simulink model "BIM_3phaseModel_MidInject_DPNV"  (R2022b)
settings: Solver=VariableStepAuto  StartTime=0.0  StopTime=3  RelTol=1e-3
values from neighbouring files (symbols this model uses):
  Ad_s1_s = 0.730402691048646    (= 0.730402691049)    [BIM_init.m]
  Ad_t_s = 0.881911378298176    (= 0.881911378298)    [BIM_init.m]
  Ap_s1_s = 0.975904794542392    (= 0.975904794542)    [BIM_init.m]
  Ap_t_s = 0.995669127615556    (= 0.995669127616)    [BIM_init.m]
  Bd_s1_s = 0.269597308951354    (= 0.269597308951)    [BIM_init.m]
  Bd_t_s = 0.118088621701824    (= 0.118088621702)    [BIM_init.m]
  Bp_s1_s = 0.269597308951354    (= 0.269597308951)    [BIM_init.m]
  Bp_t_s = 0.118088621701824    (= 0.118088621702)    [BIM_init.m]
  Ctr_v_Ki = Ctr_v_Kp*0.1    (= 0.1)    [BIM_init.m]
  Ctr_v_Kp = 1    [BIM_init.m]
  L_m = 5.02e-3    (= 0.00502)    [BIM_init.m]
  L_r = L_m + L_sigma_r    (= 0.00576)    [BIM_init.m]
  m_rotor = 1.5    [BIM_init.m]
  PolePair = 1    [BIM_init.m]
  r_s1_s = 2*R_s    (= 1)    [BIM_init.m]
  r_t_s = R_s/2    (= 0.25)    [BIM_init.m]
  T = 1/fsw    (= 0.0001)    [BIM_init.m]
  tau_r = 0.012255319148936    (= 0.0122553191489)    [BIM_init.m]
  Ts = 1/fsw    (= 0.0001)    [BIM_init.m]
undefined symbols (not defined in the file or in its folder): plecs, sigbuilder_block
libraries: spsabctodq0Lib x8, spsdq0toabcLib x4
(part 2 of 2)

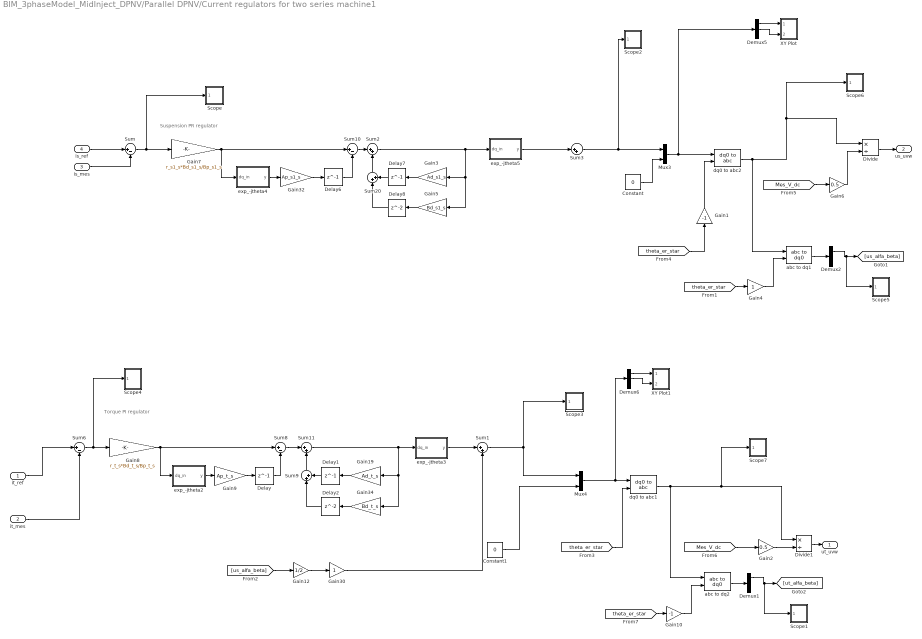
== system BIM_3phaseModel_MidInject_DPNV/Parallel DPNV/Current regulators for two series machine1 ==
  note: Suspension PR regulator
  note: Torque PI regulator
  it_ref : Inport  PortDimensions=2
  it_mes : Inport  Port=2  PortDimensions=2
  is_mes : Inport  Port=3  PortDimensions=2
  is_ref : Inport  Port=4  PortDimensions=2
  Constant : Constant  Value=0
  Constant1 : Constant  Value=0
  Delay{,1,6..7} (4 alike) : Delay  DelayLength=1  SampleTime=Ts
  Delay2 : Delay  SampleTime=Ts
  Delay8 : Delay  SampleTime=Ts
  Demux1 : Demux  Outputs=[2 1]
  Demux2 : Demux  Outputs=[2 1]
  Demux5 : Demux  Outputs=3
  Demux6 : Demux  Outputs=3
  Divide : Product  Inputs=*/
  Divide1 : Product  Inputs=*/
  Gain1 : Gain  Gain=-1
  Gain10 : Gain  Gain=-1
  Gain12 : Gain  Gain=1/2
  Gain19 : Gain  Gain=Ad_t_s
  Gain2 : Gain  Gain=0.5
  Gain3 : Gain  Gain=Ad_s1_s
  Gain30 : Gain
  Gain32 : Gain  Gain=Ap_s1_s
  Gain34 : Gain  Gain=Bd_t_s
  Gain4 : Gain
  Gain5 : Gain  Gain=Bd_s1_s
  Gain6 : Gain  Gain=0.5
  Gain7 : Gain  Gain=r_s1_s*Bd_s1_s/Bp_s1_s
  Gain8 : Gain  Gain=r_t_s*Bd_t_s/Bp_t_s
  Gain9 : Gain  Gain=Ap_t_s
  Mux3 : Mux  Inputs=[2 1]
  Mux4 : Mux  Inputs=[2 1]
  Scope : Subsystem  LoadFcn=plecs('sl', 300);  InitFcn=plecs('sl', 314);  StartFcn=plecs('sl', 308);  StopFcn=plecs('sl', 309);  mask{Settings=<binary blob, 232 chars, not shown>}
      mask init:
      | plecs('sl', 315);
      settings: CopyFcn=plecs('sl', 303);  DeleteFcn=plecs('sl', 305);  UndoDeleteFcn=plecs('sl', 306);  PreSaveFcn=plecs('sl', 311);  NameChangeFcn=plecs('sl', 310);  DestroyFcn=plecs('sl', 307);  OpenFcn=plecs('sl', 302);  ErrorFcn=plerrorfcn
      mask Display: plot([0.1 0.9 0.9 0.1 0.1], [0.9 0.9 0.5 0.5 0.9])
  Scope1 : Subsystem  LoadFcn=plecs('sl', 300);  InitFcn=plecs('sl', 314);  StartFcn=plecs('sl', 308);  StopFcn=plecs('sl', 309);  mask{Settings=<binary blob, 232 chars, not shown>}
      mask init:
      | plecs('sl', 315);
      settings: CopyFcn=plecs('sl', 303);  DeleteFcn=plecs('sl', 305);  UndoDeleteFcn=plecs('sl', 306);  PreSaveFcn=plecs('sl', 311);  NameChangeFcn=plecs('sl', 310);  DestroyFcn=plecs('sl', 307);  OpenFcn=plecs('sl', 302);  ErrorFcn=plerrorfcn
      mask Display: plot([0.1 0.9 0.9 0.1 0.1], [0.9 0.9 0.5 0.5 0.9])
  Scope2 : Subsystem  LoadFcn=plecs('sl', 300);  InitFcn=plecs('sl', 314);  StartFcn=plecs('sl', 308);  StopFcn=plecs('sl', 309);  mask{Settings=<binary blob, 232 chars, not shown>}
      mask init:
      | plecs('sl', 315);
      settings: CopyFcn=plecs('sl', 303);  DeleteFcn=plecs('sl', 305);  UndoDeleteFcn=plecs('sl', 306);  PreSaveFcn=plecs('sl', 311);  NameChangeFcn=plecs('sl', 310);  DestroyFcn=plecs('sl', 307);  OpenFcn=plecs('sl', 302);  ErrorFcn=plerrorfcn
      mask Display: plot([0.1 0.9 0.9 0.1 0.1], [0.9 0.9 0.5 0.5 0.9])
  Scope3 : Subsystem  LoadFcn=plecs('sl', 300);  InitFcn=plecs('sl', 314);  StartFcn=plecs('sl', 308);  StopFcn=plecs('sl', 309);  mask{Settings=<binary blob, 232 chars, not shown>}
      mask init:
      | plecs('sl', 315);
      settings: CopyFcn=plecs('sl', 303);  DeleteFcn=plecs('sl', 305);  UndoDeleteFcn=plecs('sl', 306);  PreSaveFcn=plecs('sl', 311);  NameChangeFcn=plecs('sl', 310);  DestroyFcn=plecs('sl', 307);  OpenFcn=plecs('sl', 302);  ErrorFcn=plerrorfcn
      mask Display: plot([0.1 0.9 0.9 0.1 0.1], [0.9 0.9 0.5 0.5 0.9])
  Scope4 : Subsystem  LoadFcn=plecs('sl', 300);  InitFcn=plecs('sl', 314);  StartFcn=plecs('sl', 308);  StopFcn=plecs('sl', 309);  mask{Settings=<binary blob, 232 chars, not shown>}
      mask init:
      | plecs('sl', 315);
      settings: CopyFcn=plecs('sl', 303);  DeleteFcn=plecs('sl', 305);  UndoDeleteFcn=plecs('sl', 306);  PreSaveFcn=plecs('sl', 311);  NameChangeFcn=plecs('sl', 310);  DestroyFcn=plecs('sl', 307);  OpenFcn=plecs('sl', 302);  ErrorFcn=plerrorfcn
      mask Display: plot([0.1 0.9 0.9 0.1 0.1], [0.9 0.9 0.5 0.5 0.9])
  Scope5 : Subsystem  LoadFcn=plecs('sl', 300);  InitFcn=plecs('sl', 314);  StartFcn=plecs('sl', 308);  StopFcn=plecs('sl', 309);  mask{Settings=<binary blob, 232 chars, not shown>}
      mask init:
      | plecs('sl', 315);
      settings: CopyFcn=plecs('sl', 303);  DeleteFcn=plecs('sl', 305);  UndoDeleteFcn=plecs('sl', 306);  PreSaveFcn=plecs('sl', 311);  NameChangeFcn=plecs('sl', 310);  DestroyFcn=plecs('sl', 307);  OpenFcn=plecs('sl', 302);  ErrorFcn=plerrorfcn
      mask Display: plot([0.1 0.9 0.9 0.1 0.1], [0.9 0.9 0.5 0.5 0.9])
  Scope6 : Subsystem  LoadFcn=plecs('sl', 300);  InitFcn=plecs('sl', 314);  StartFcn=plecs('sl', 308);  StopFcn=plecs('sl', 309);  mask{Settings=<binary blob, 232 chars, not shown>}
      mask init:
      | plecs('sl', 315);
      settings: CopyFcn=plecs('sl', 303);  DeleteFcn=plecs('sl', 305);  UndoDeleteFcn=plecs('sl', 306);  PreSaveFcn=plecs('sl', 311);  NameChangeFcn=plecs('sl', 310);  DestroyFcn=plecs('sl', 307);  OpenFcn=plecs('sl', 302);  ErrorFcn=plerrorfcn
      mask Display: plot([0.1 0.9 0.9 0.1 0.1], [0.9 0.9 0.5 0.5 0.9])
  Scope7 : Subsystem  LoadFcn=plecs('sl', 300);  InitFcn=plecs('sl', 314);  StartFcn=plecs('sl', 308);  StopFcn=plecs('sl', 309);  mask{Settings=<binary blob, 232 chars, not shown>}
      mask init:
      | plecs('sl', 315);
      settings: CopyFcn=plecs('sl', 303);  DeleteFcn=plecs('sl', 305);  UndoDeleteFcn=plecs('sl', 306);  PreSaveFcn=plecs('sl', 311);  NameChangeFcn=plecs('sl', 310);  DestroyFcn=plecs('sl', 307);  OpenFcn=plecs('sl', 302);  ErrorFcn=plerrorfcn
      mask Display: plot([0.1 0.9 0.9 0.1 0.1], [0.9 0.9 0.5 0.5 0.9])
  Sum{,6,8,10} (4 alike) : Sum  Inputs=|+-
  Sum{1..3,9,11,20} (6 alike) : Sum  Inputs=|++
  XY Plot : Subsystem  LoadFcn=plecs('sl', 317);  InitFcn=plecs('sl', 314);  StartFcn=plecs('sl', 308);  StopFcn=plecs('sl', 309);  mask{Settings=<binary blob, 240 chars, not shown>}
      mask init:
      | plecs('sl', 315);
      settings: CopyFcn=plecs('sl', 318);  DeleteFcn=plecs('sl', 305);  UndoDeleteFcn=plecs('sl', 306);  PreSaveFcn=plecs('sl', 311);  NameChangeFcn=plecs('sl', 310);  DestroyFcn=plecs('sl', 307);  OpenFcn=plecs('sl', 302);  ErrorFcn=plerrorfcn
      mask Display:
      | plot([0.05 0.95 0.95 0.05 0.05], [0.95 0.95 0.05 0.05 0.95])
      | plot(0.5+sin((0:0.2:2)*pi)*0.3, 0.5+sin((0:0.2:2)*pi + pi/4)*0.3);
  XY Plot1 : Subsystem  LoadFcn=plecs('sl', 317);  InitFcn=plecs('sl', 314);  StartFcn=plecs('sl', 308);  StopFcn=plecs('sl', 309);  mask{Settings=<binary blob, 240 chars, not shown>}
      mask init:
      | plecs('sl', 315);
      settings: CopyFcn=plecs('sl', 318);  DeleteFcn=plecs('sl', 305);  UndoDeleteFcn=plecs('sl', 306);  PreSaveFcn=plecs('sl', 311);  NameChangeFcn=plecs('sl', 310);  DestroyFcn=plecs('sl', 307);  OpenFcn=plecs('sl', 302);  ErrorFcn=plerrorfcn
      mask Display:
      | plot([0.05 0.95 0.95 0.05 0.05], [0.95 0.95 0.05 0.05 0.95])
      | plot(0.5+sin((0:0.2:2)*pi)*0.3, 0.5+sin((0:0.2:2)*pi + pi/4)*0.3);
  abc to dq1 : spsabctodq0Lib/abc to dq0  Alignment=Aligned with phase A axis
  abc to dq2 : spsabctodq0Lib/abc to dq0  Alignment=Aligned with phase A axis
  dq0 to abc1 : spsdq0toabcLib/dq0 to abc  Alignment=Aligned with phase A axis
  dq0 to abc2 : spsdq0toabcLib/dq0 to abc  Alignment=Aligned with phase A axis
  exp_-jtheta2 : Subsystem
  exp_-jtheta3 : Subsystem
  exp_-jtheta4 : Subsystem
  exp_-jtheta5 : Subsystem
  ut_uvw : Outport  PortDimensions=3
  us_uvw : Outport  Port=2  PortDimensions=3
  wires:
  Sum6/1 -> Scope4/1(1), Gain8/1
  Mux3/1 -> Demux5/1, dq0 to abc2/1
  dq0 to abc2/1 -> abc to dq1/1, Divide/1, Scope6/1(1)
  Sum11/1 -> Gain34/1, Gain19/1, exp_-jtheta3/1(dq_in)
  Constant1/1 -> Mux4/2
  Demux5/1 -> XY Plot/1(1)
  Demux5/2 -> XY Plot/2(2)
  Demux6/2 -> XY Plot1/2(2)
  Demux6/1 -> XY Plot1/1(1)
  Constant/1 -> Mux3/2
  Gain8/1 -> Sum8/1, exp_-jtheta2/1(dq_in)
  Gain9/1 -> Delay/1
  Sum8/1 -> Sum11/1
  Delay/1 -> Sum8/2
  Gain19/1 -> Delay1/1
  Gain34/1 -> Delay2/1
  Delay1/1 -> Sum9/2
  Delay2/1 -> Sum9/1
  Sum9/1 -> Sum11/2
  Sum2/1 -> Gain5/1, Gain3/1, exp_-jtheta5/1(dq_in)
  Delay8/1 -> Sum20/1
  Delay7/1 -> Sum20/2
  Delay6/1 -> Sum10/2
  Gain5/1 -> Delay8/1
  Sum20/1 -> Sum2/2
  Gain3/1 -> Delay7/1
  Sum/1 -> Gain7/1, Scope/1(1)
  Gain32/1 -> Delay6/1
  Gain7/1 -> Sum10/1, exp_-jtheta4/1(dq_in)
  Sum10/1 -> Sum2/1
  it_ref/1 -> Sum6/1
  it_mes/1 -> Sum6/2
  exp_-jtheta2/1(y) -> Gain9/1
  [theta_er_star] -> dq0 to abc1/2
  is_ref/1 -> Sum/1
  is_mes/1 -> Sum/2
  exp_-jtheta4/1(y) -> Gain32/1
  [theta_er_star] -> Gain1/1
  Gain1/1 -> dq0 to abc2/2
  abc to dq1/1 -> Demux2/1
  [theta_er_star] -> Gain4/1
  Gain4/1 -> abc to dq1/2
  Demux2/1 -> Scope5/1(1), [us_alfa_beta]
  Gain12/1 -> Gain30/1
  [us_alfa_beta] -> Gain12/1
  exp_-jtheta3/1(y) -> Sum1/1
  [Mes_V_dc] -> Gain6/1
  Divide/1 -> us_uvw/1
  [Mes_V_dc] -> Gain2/1
  Divide1/1 -> ut_uvw/1
  Gain2/1 -> Divide1/2
  Gain6/1 -> Divide/2
  Demux1/1 -> Scope1/1(1), [ut_alfa_beta]
  [theta_er_star] -> Gain10/1
  Gain10/1 -> abc to dq2/2
  dq0 to abc1/1 -> abc to dq2/1, Scope7/1(1), Divide1/1
  abc to dq2/1 -> Demux1/1
  Mux4/1 -> Demux6/1, dq0 to abc1/1
  Sum1/1 -> Mux4/1, Scope3/1(1)
  Sum3/1 -> Scope2/1(1), Mux3/1
  exp_-jtheta5/1(y) -> Sum3/1
  Gain30/1 -> Sum1/2

== system BIM_3phaseModel_MidInject_DPNV/Parallel DPNV/Scope1 ==
  1 : Inport
  2 : Inport  Port=2
  " 1 " : DataTypeConversion
  " 2 " : DataTypeConversion
  " InputMux " : Mux  Inputs=2
  " S-Function " : S-Function  FunctionName=plecs  SFunctionDeploymentMode=off  EnableBusSupport=off
  wires:
  " InputMux "/1 -> " S-Function "/1
  1/1 -> " 1 "/1
  " 1 "/1 -> " InputMux "/1
  2/1 -> " 2 "/1
  " 2 "/1 -> " InputMux "/2

== system BIM_3phaseModel_MidInject_DPNV/Parallel DPNV/Scope13 ==
  1 : Inport
  " 1 " : DataTypeConversion
  " InputMux " : Mux  Inputs=1
  " S-Function " : S-Function  FunctionName=plecs  SFunctionDeploymentMode=off  EnableBusSupport=off
  wires:
  " InputMux "/1 -> " S-Function "/1
  1/1 -> " 1 "/1
  " 1 "/1 -> " InputMux "/1

== system BIM_3phaseModel_MidInject_DPNV/Parallel DPNV/Scope15 ==
  1 : Inport
  2 : Inport  Port=2
  " 1 " : DataTypeConversion
  " 2 " : DataTypeConversion
  " InputMux " : Mux  Inputs=2
  " S-Function " : S-Function  FunctionName=plecs  SFunctionDeploymentMode=off  EnableBusSupport=off
  wires:
  " InputMux "/1 -> " S-Function "/1
  1/1 -> " 1 "/1
  " 1 "/1 -> " InputMux "/1
  2/1 -> " 2 "/1
  " 2 "/1 -> " InputMux "/2

== system BIM_3phaseModel_MidInject_DPNV/Parallel DPNV/Scope16 ==
  1 : Inport
  " 1 " : DataTypeConversion
  " InputMux " : Mux  Inputs=1
  " S-Function " : S-Function  FunctionName=plecs  SFunctionDeploymentMode=off  EnableBusSupport=off
  wires:
  " InputMux "/1 -> " S-Function "/1
  1/1 -> " 1 "/1
  " 1 "/1 -> " InputMux "/1

== system BIM_3phaseModel_MidInject_DPNV/Parallel DPNV/Scope17 ==
  1 : Inport
  2 : Inport  Port=2
  3 : Inport  Port=3
  " 1 " : DataTypeConversion
  " 2 " : DataTypeConversion
  " 3 " : DataTypeConversion
  " InputMux " : Mux  Inputs=3
  " S-Function " : S-Function  FunctionName=plecs  SFunctionDeploymentMode=off  EnableBusSupport=off
  wires:
  " InputMux "/1 -> " S-Function "/1
  1/1 -> " 1 "/1
  " 1 "/1 -> " InputMux "/1
  2/1 -> " 2 "/1
  " 2 "/1 -> " InputMux "/2
  3/1 -> " 3 "/1
  " 3 "/1 -> " InputMux "/3

== system BIM_3phaseModel_MidInject_DPNV/Parallel DPNV/Scope18 ==
  1 : Inport
  2 : Inport  Port=2
  3 : Inport  Port=3
  " 1 " : DataTypeConversion
  " 2 " : DataTypeConversion
  " 3 " : DataTypeConversion
  " InputMux " : Mux  Inputs=3
  " S-Function " : S-Function  FunctionName=plecs  SFunctionDeploymentMode=off  EnableBusSupport=off
  wires:
  " InputMux "/1 -> " S-Function "/1
  1/1 -> " 1 "/1
  " 1 "/1 -> " InputMux "/1
  2/1 -> " 2 "/1
  " 2 "/1 -> " InputMux "/2
  3/1 -> " 3 "/1
  " 3 "/1 -> " InputMux "/3

== system BIM_3phaseModel_MidInject_DPNV/Parallel DPNV/Scope4 ==
  1 : Inport
  " 1 " : DataTypeConversion
  " InputMux " : Mux  Inputs=1
  " S-Function " : S-Function  FunctionName=plecs  SFunctionDeploymentMode=off  EnableBusSupport=off
  wires:
  " InputMux "/1 -> " S-Function "/1
  1/1 -> " 1 "/1
  " 1 "/1 -> " InputMux "/1

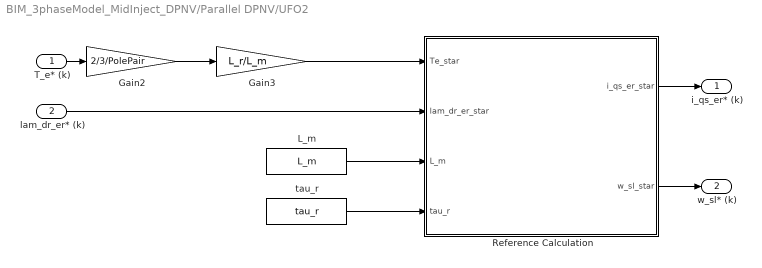
== system BIM_3phaseModel_MidInject_DPNV/Parallel DPNV/UFO2 ==
  T_e* (k) : Inport
  lam_dr_er* (k) : Inport  Port=2
  Gain2 : Gain  Gain=2/3/PolePair
  Gain3 : Gain  Gain=L_r/L_m
  L_m : Constant  Value=L_m
  Reference Calculation : MATLAB Function  TreatAsAtomicUnit=on
  tau_r : Constant  Value=tau_r
  i_qs_er* (k) : Outport
  w_sl* (k) : Outport  Port=2
  wires:
  lam_dr_er* (k)/1 -> Reference Calculation/2(lam_dr_er_star)
  T_e* (k)/1 -> Gain2/1
  Gain2/1 -> Gain3/1
  Gain3/1 -> Reference Calculation/1(Te_star)
  L_m/1 -> Reference Calculation/3(L_m)
  tau_r/1 -> Reference Calculation/4(tau_r)
  Reference Calculation/2(w_sl_star) -> w_sl* (k)/1
  Reference Calculation/1(i_qs_er_star) -> i_qs_er* (k)/1

== system BIM_3phaseModel_MidInject_DPNV/Parallel DPNV/Velocity Regulator ==
  w_rm* (k) : Inport
  w_rm (k) : Inport  Port=2
  Rate Limiter : RateLimiter  RisingSlewLimit=50  FallingSlewLimit=-50  SampleTimeMode=inherited
  Scope4 : Subsystem  LoadFcn=plecs('sl', 300);  InitFcn=plecs('sl', 314);  StartFcn=plecs('sl', 308);  StopFcn=plecs('sl', 309);  mask{Settings=<binary blob, 232 chars, not shown>}
      mask init:
      | plecs('sl', 315);
      settings: CopyFcn=plecs('sl', 303);  DeleteFcn=plecs('sl', 305);  UndoDeleteFcn=plecs('sl', 306);  PreSaveFcn=plecs('sl', 311);  NameChangeFcn=plecs('sl', 310);  DestroyFcn=plecs('sl', 307);  OpenFcn=plecs('sl', 302);  ErrorFcn=plerrorfcn
      mask Display: plot([0.1 0.9 0.9 0.1 0.1], [0.9 0.9 0.5 0.5 0.9])
  Sum : Sum  Inputs=|+-
  velocity regulator : Subsystem
  Te* (k) : Outport  PortDimensions=1
  wires:
  Sum/1 -> Scope4/1(1), velocity regulator/1(Err_v)
  w_rm (k)/1 -> Sum/2
  velocity regulator/1(Te*) -> Scope4/2(2), Te* (k)/1
  w_rm* (k)/1 -> Rate Limiter/1
  Rate Limiter/1 -> Sum/1

== system BIM_3phaseModel_MidInject_DPNV/Parallel DPNV/XY Plot1 ==
  1 : Inport
  2 : Inport  Port=2
  " InputMux " : Subsystem
      mask Display: disp('Mux')
  " S-Function " : S-Function  FunctionName=plecs  SFunctionDeploymentMode=off  EnableBusSupport=off
  wires:
  2/1 -> " InputMux "/1(In1)
  1/1 -> " InputMux "/2(In2)
  " InputMux "/1(Out) -> " S-Function "/1

== system BIM_3phaseModel_MidInject_DPNV/Mid Injection/CFO/Scope1 ==
  1 : Inport
  2 : Inport  Port=2
  3 : Inport  Port=3
  " 1 " : DataTypeConversion
  " 2 " : DataTypeConversion
  " 3 " : DataTypeConversion
  " InputMux " : Mux  Inputs=3
  " S-Function " : S-Function  FunctionName=plecs  SFunctionDeploymentMode=off  EnableBusSupport=off
  wires:
  " InputMux "/1 -> " S-Function "/1
  1/1 -> " 1 "/1
  " 1 "/1 -> " InputMux "/1
  2/1 -> " 2 "/1
  " 2 "/1 -> " InputMux "/2
  3/1 -> " 3 "/1
  " 3 "/1 -> " InputMux "/3

== system BIM_3phaseModel_MidInject_DPNV/Mid Injection/CFO/Scope8 ==
  1 : Inport
  2 : Inport  Port=2
  3 : Inport  Port=3
  " 1 " : DataTypeConversion
  " 2 " : DataTypeConversion
  " 3 " : DataTypeConversion
  " InputMux " : Mux  Inputs=3
  " S-Function " : S-Function  FunctionName=plecs  SFunctionDeploymentMode=off  EnableBusSupport=off
  wires:
  " InputMux "/1 -> " S-Function "/1
  1/1 -> " 1 "/1
  " 1 "/1 -> " InputMux "/1
  2/1 -> " 2 "/1
  " 2 "/1 -> " InputMux "/2
  3/1 -> " 3 "/1
  " 3 "/1 -> " InputMux "/3

== system BIM_3phaseModel_MidInject_DPNV/Mid Injection/Current regulators for two series machine1/Scope ==
  1 : Inport
  " InputMux " : Subsystem
      mask Display: disp('Mux')
  " S-Function " : S-Function  FunctionName=plecs  SFunctionDeploymentMode=off  EnableBusSupport=off
  wires:
  1/1 -> " InputMux "/1(In1)
  " InputMux "/1(Out) -> " S-Function "/1

== system BIM_3phaseModel_MidInject_DPNV/Mid Injection/Current regulators for two series machine1/Scope1 ==
  1 : Inport
  " InputMux " : Subsystem
      mask Display: disp('Mux')
  " S-Function " : S-Function  FunctionName=plecs  SFunctionDeploymentMode=off  EnableBusSupport=off
  wires:
  1/1 -> " InputMux "/1(In1)
  " InputMux "/1(Out) -> " S-Function "/1

== system BIM_3phaseModel_MidInject_DPNV/Mid Injection/Current regulators for two series machine1/Scope2 ==
  1 : Inport
  " InputMux " : Subsystem
      mask Display: disp('Mux')
  " S-Function " : S-Function  FunctionName=plecs  SFunctionDeploymentMode=off  EnableBusSupport=off
  wires:
  1/1 -> " InputMux "/1(In1)
  " InputMux "/1(Out) -> " S-Function "/1

== system BIM_3phaseModel_MidInject_DPNV/Mid Injection/Current regulators for two series machine1/Scope3 ==
  1 : Inport
  " InputMux " : Subsystem
      mask Display: disp('Mux')
  " S-Function " : S-Function  FunctionName=plecs  SFunctionDeploymentMode=off  EnableBusSupport=off
  wires:
  1/1 -> " InputMux "/1(In1)
  " InputMux "/1(Out) -> " S-Function "/1

== system BIM_3phaseModel_MidInject_DPNV/Mid Injection/Current regulators for two series machine1/Scope4 ==
  1 : Inport
  " 1 " : DataTypeConversion
  " InputMux " : Mux  Inputs=1
  " S-Function " : S-Function  FunctionName=plecs  SFunctionDeploymentMode=off  EnableBusSupport=off
  wires:
  " InputMux "/1 -> " S-Function "/1
  1/1 -> " 1 "/1
  " 1 "/1 -> " InputMux "/1

== system BIM_3phaseModel_MidInject_DPNV/Mid Injection/Current regulators for two series machine1/Scope5 ==
  1 : Inport
  " InputMux " : Subsystem
      mask Display: disp('Mux')
  " S-Function " : S-Function  FunctionName=plecs  SFunctionDeploymentMode=off  EnableBusSupport=off
  wires:
  1/1 -> " InputMux "/1(In1)
  " InputMux "/1(Out) -> " S-Function "/1

== system BIM_3phaseModel_MidInject_DPNV/Mid Injection/Current regulators for two series machine1/Scope6 ==
  1 : Inport
  " InputMux " : Subsystem
      mask Display: disp('Mux')
  " S-Function " : S-Function  FunctionName=plecs  SFunctionDeploymentMode=off  EnableBusSupport=off
  wires:
  1/1 -> " InputMux "/1(In1)
  " InputMux "/1(Out) -> " S-Function "/1

== system BIM_3phaseModel_MidInject_DPNV/Mid Injection/Current regulators for two series machine1/Scope7 ==
  1 : Inport
  " InputMux " : Subsystem
      mask Display: disp('Mux')
  " S-Function " : S-Function  FunctionName=plecs  SFunctionDeploymentMode=off  EnableBusSupport=off
  wires:
  1/1 -> " InputMux "/1(In1)
  " InputMux "/1(Out) -> " S-Function "/1

== system BIM_3phaseModel_MidInject_DPNV/Mid Injection/Current regulators for two series machine1/XY Plot ==
  1 : Inport
  2 : Inport  Port=2
  " InputMux " : Subsystem
      mask Display: disp('Mux')
  " S-Function " : S-Function  FunctionName=plecs  SFunctionDeploymentMode=off  EnableBusSupport=off
  wires:
  2/1 -> " InputMux "/1(In1)
  1/1 -> " InputMux "/2(In2)
  " InputMux "/1(Out) -> " S-Function "/1

== system BIM_3phaseModel_MidInject_DPNV/Mid Injection/Current regulators for two series machine1/XY Plot1 ==
  1 : Inport
  2 : Inport  Port=2
  " InputMux " : Subsystem
      mask Display: disp('Mux')
  " S-Function " : S-Function  FunctionName=plecs  SFunctionDeploymentMode=off  EnableBusSupport=off
  wires:
  2/1 -> " InputMux "/1(In1)
  1/1 -> " InputMux "/2(In2)
  " InputMux "/1(Out) -> " S-Function "/1

== system BIM_3phaseModel_MidInject_DPNV/Mid Injection/Current regulators for two series machine1/exp_-jtheta2 ==
  dq_in : Inport
  Gain : Gain  Gain=-Ts
  Gain1 : Gain
  MATLAB Function : MATLAB Function  TreatAsAtomicUnit=on
  y : Outport  PortDimensions=2
  wires:
  dq_in/1 -> MATLAB Function/1(u_dq)
  [w_e] -> Gain1/1
  Gain/1 -> MATLAB Function/2(theta)
  MATLAB Function/1(y) -> y/1
  Gain1/1 -> Gain/1

== system BIM_3phaseModel_MidInject_DPNV/Mid Injection/Current regulators for two series machine1/exp_-jtheta3 ==
  dq_in : Inport
  Gain : Gain  Gain=2*Ts
  Gain1 : Gain
  MATLAB Function : MATLAB Function  TreatAsAtomicUnit=on
  y : Outport  PortDimensions=2
  wires:
  dq_in/1 -> MATLAB Function/1(u_dq)
  [w_e] -> Gain1/1
  Gain/1 -> MATLAB Function/2(theta)
  MATLAB Function/1(y) -> y/1
  Gain1/1 -> Gain/1

== system BIM_3phaseModel_MidInject_DPNV/Mid Injection/Current regulators for two series machine1/exp_-jtheta4 ==
  dq_in : Inport
  Gain : Gain  Gain=-Ts
  Gain1 : Gain  Gain=-1
  MATLAB Function : MATLAB Function  TreatAsAtomicUnit=on
  y : Outport  PortDimensions=2
  wires:
  dq_in/1 -> MATLAB Function/1(u_dq)
  [w_e] -> Gain1/1
  Gain/1 -> MATLAB Function/2(theta)
  MATLAB Function/1(y) -> y/1
  Gain1/1 -> Gain/1

== system BIM_3phaseModel_MidInject_DPNV/Mid Injection/Current regulators for two series machine1/exp_-jtheta5 ==
  dq_in : Inport
  Gain : Gain  Gain=2*Ts
  Gain1 : Gain  Gain=-1
  MATLAB Function : MATLAB Function  TreatAsAtomicUnit=on
  y : Outport  PortDimensions=2
  wires:
  dq_in/1 -> MATLAB Function/1(u_dq)
  [w_e] -> Gain1/1
  Gain/1 -> MATLAB Function/2(theta)
  MATLAB Function/1(y) -> y/1
  Gain1/1 -> Gain/1

== system BIM_3phaseModel_MidInject_DPNV/Mid Injection/Velocity Regulator/Scope4 ==
  1 : Inport
  2 : Inport  Port=2
  " 1 " : DataTypeConversion
  " 2 " : DataTypeConversion
  " InputMux " : Mux  Inputs=2
  " S-Function " : S-Function  FunctionName=plecs  SFunctionDeploymentMode=off  EnableBusSupport=off
  wires:
  " InputMux "/1 -> " S-Function "/1
  1/1 -> " 1 "/1
  " 1 "/1 -> " InputMux "/1
  2/1 -> " 2 "/1
  " 2 "/1 -> " InputMux "/2

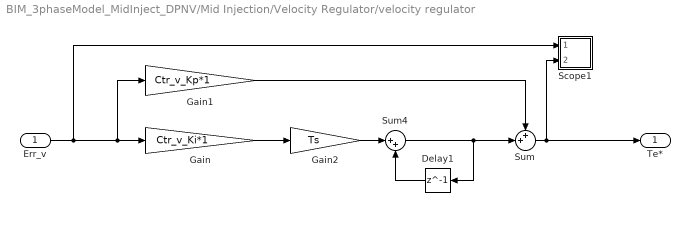
== system BIM_3phaseModel_MidInject_DPNV/Mid Injection/Velocity Regulator/velocity regulator ==
  Err_v : Inport
  Delay1 : Delay  DelayLength=1  SampleTime=T
  Gain : Gain  Gain=Ctr_v_Ki*1
  Gain1 : Gain  Gain=Ctr_v_Kp*1
  Gain2 : Gain  Gain=Ts
  Scope1 : Subsystem  LoadFcn=plecs('sl', 300);  InitFcn=plecs('sl', 314);  StartFcn=plecs('sl', 308);  StopFcn=plecs('sl', 309);  mask{Settings=<binary blob, 232 chars, not shown>}
      mask init:
      | plecs('sl', 315);
      settings: CopyFcn=plecs('sl', 303);  DeleteFcn=plecs('sl', 305);  UndoDeleteFcn=plecs('sl', 306);  PreSaveFcn=plecs('sl', 311);  NameChangeFcn=plecs('sl', 310);  DestroyFcn=plecs('sl', 307);  OpenFcn=plecs('sl', 302);  ErrorFcn=plerrorfcn
      mask Display: plot([0.1 0.9 0.9 0.1 0.1], [0.9 0.9 0.5 0.5 0.9])
  Sum : Sum  Inputs=++|
  Sum4 : Sum  Inputs=|++
  Te* : Outport
  wires:
  Err_v/1 -> Scope1/1(1), Gain1/1, Gain/1
  Gain1/1 -> Sum/1
  Sum/1 -> Scope1/2(2), Te*/1
  Gain2/1 -> Sum4/1
  Gain/1 -> Gain2/1
  Sum4/1 -> Delay1/1, Sum/2
  Delay1/1 -> Sum4/2

== system BIM_3phaseModel_MidInject_DPNV/Parallel DPNV/CFO/Scope1 ==
  1 : Inport
  2 : Inport  Port=2
  3 : Inport  Port=3
  " 1 " : DataTypeConversion
  " 2 " : DataTypeConversion
  " 3 " : DataTypeConversion
  " InputMux " : Mux  Inputs=3
  " S-Function " : S-Function  FunctionName=plecs  SFunctionDeploymentMode=off  EnableBusSupport=off
  wires:
  " InputMux "/1 -> " S-Function "/1
  1/1 -> " 1 "/1
  " 1 "/1 -> " InputMux "/1
  2/1 -> " 2 "/1
  " 2 "/1 -> " InputMux "/2
  3/1 -> " 3 "/1
  " 3 "/1 -> " InputMux "/3

== system BIM_3phaseModel_MidInject_DPNV/Parallel DPNV/CFO/Scope8 ==
  1 : Inport
  2 : Inport  Port=2
  3 : Inport  Port=3
  " 1 " : DataTypeConversion
  " 2 " : DataTypeConversion
  " 3 " : DataTypeConversion
  " InputMux " : Mux  Inputs=3
  " S-Function " : S-Function  FunctionName=plecs  SFunctionDeploymentMode=off  EnableBusSupport=off
  wires:
  " InputMux "/1 -> " S-Function "/1
  1/1 -> " 1 "/1
  " 1 "/1 -> " InputMux "/1
  2/1 -> " 2 "/1
  " 2 "/1 -> " InputMux "/2
  3/1 -> " 3 "/1
  " 3 "/1 -> " InputMux "/3

== system BIM_3phaseModel_MidInject_DPNV/Parallel DPNV/Current regulators for two series machine1/Scope ==
  1 : Inport
  " InputMux " : Subsystem
      mask Display: disp('Mux')
  " S-Function " : S-Function  FunctionName=plecs  SFunctionDeploymentMode=off  EnableBusSupport=off
  wires:
  1/1 -> " InputMux "/1(In1)
  " InputMux "/1(Out) -> " S-Function "/1

== system BIM_3phaseModel_MidInject_DPNV/Parallel DPNV/Current regulators for two series machine1/Scope1 ==
  1 : Inport
  " InputMux " : Subsystem
      mask Display: disp('Mux')
  " S-Function " : S-Function  FunctionName=plecs  SFunctionDeploymentMode=off  EnableBusSupport=off
  wires:
  1/1 -> " InputMux "/1(In1)
  " InputMux "/1(Out) -> " S-Function "/1

== system BIM_3phaseModel_MidInject_DPNV/Parallel DPNV/Current regulators for two series machine1/Scope2 ==
  1 : Inport
  " InputMux " : Subsystem
      mask Display: disp('Mux')
  " S-Function " : S-Function  FunctionName=plecs  SFunctionDeploymentMode=off  EnableBusSupport=off
  wires:
  1/1 -> " InputMux "/1(In1)
  " InputMux "/1(Out) -> " S-Function "/1

== system BIM_3phaseModel_MidInject_DPNV/Parallel DPNV/Current regulators for two series machine1/Scope3 ==
  1 : Inport
  " InputMux " : Subsystem
      mask Display: disp('Mux')
  " S-Function " : S-Function  FunctionName=plecs  SFunctionDeploymentMode=off  EnableBusSupport=off
  wires:
  1/1 -> " InputMux "/1(In1)
  " InputMux "/1(Out) -> " S-Function "/1

== system BIM_3phaseModel_MidInject_DPNV/Parallel DPNV/Current regulators for two series machine1/Scope4 ==
  1 : Inport
  " 1 " : DataTypeConversion
  " InputMux " : Mux  Inputs=1
  " S-Function " : S-Function  FunctionName=plecs  SFunctionDeploymentMode=off  EnableBusSupport=off
  wires:
  " InputMux "/1 -> " S-Function "/1
  1/1 -> " 1 "/1
  " 1 "/1 -> " InputMux "/1

== system BIM_3phaseModel_MidInject_DPNV/Parallel DPNV/Current regulators for two series machine1/Scope5 ==
  1 : Inport
  " InputMux " : Subsystem
      mask Display: disp('Mux')
  " S-Function " : S-Function  FunctionName=plecs  SFunctionDeploymentMode=off  EnableBusSupport=off
  wires:
  1/1 -> " InputMux "/1(In1)
  " InputMux "/1(Out) -> " S-Function "/1

== system BIM_3phaseModel_MidInject_DPNV/Parallel DPNV/Current regulators for two series machine1/Scope6 ==
  1 : Inport
  " InputMux " : Subsystem
      mask Display: disp('Mux')
  " S-Function " : S-Function  FunctionName=plecs  SFunctionDeploymentMode=off  EnableBusSupport=off
  wires:
  1/1 -> " InputMux "/1(In1)
  " InputMux "/1(Out) -> " S-Function "/1

== system BIM_3phaseModel_MidInject_DPNV/Parallel DPNV/Current regulators for two series machine1/Scope7 ==
  1 : Inport
  " InputMux " : Subsystem
      mask Display: disp('Mux')
  " S-Function " : S-Function  FunctionName=plecs  SFunctionDeploymentMode=off  EnableBusSupport=off
  wires:
  1/1 -> " InputMux "/1(In1)
  " InputMux "/1(Out) -> " S-Function "/1

== system BIM_3phaseModel_MidInject_DPNV/Parallel DPNV/Current regulators for two series machine1/XY Plot ==
  1 : Inport
  2 : Inport  Port=2
  " InputMux " : Subsystem
      mask Display: disp('Mux')
  " S-Function " : S-Function  FunctionName=plecs  SFunctionDeploymentMode=off  EnableBusSupport=off
  wires:
  2/1 -> " InputMux "/1(In1)
  1/1 -> " InputMux "/2(In2)
  " InputMux "/1(Out) -> " S-Function "/1

== system BIM_3phaseModel_MidInject_DPNV/Parallel DPNV/Current regulators for two series machine1/XY Plot1 ==
  1 : Inport
  2 : Inport  Port=2
  " InputMux " : Subsystem
      mask Display: disp('Mux')
  " S-Function " : S-Function  FunctionName=plecs  SFunctionDeploymentMode=off  EnableBusSupport=off
  wires:
  2/1 -> " InputMux "/1(In1)
  1/1 -> " InputMux "/2(In2)
  " InputMux "/1(Out) -> " S-Function "/1

== system BIM_3phaseModel_MidInject_DPNV/Parallel DPNV/Current regulators for two series machine1/exp_-jtheta2 ==
  dq_in : Inport
  Gain : Gain  Gain=-Ts
  Gain1 : Gain
  MATLAB Function : MATLAB Function  TreatAsAtomicUnit=on
  y : Outport  PortDimensions=2
  wires:
  dq_in/1 -> MATLAB Function/1(u_dq)
  [w_e] -> Gain1/1
  Gain/1 -> MATLAB Function/2(theta)
  MATLAB Function/1(y) -> y/1
  Gain1/1 -> Gain/1

== system BIM_3phaseModel_MidInject_DPNV/Parallel DPNV/Current regulators for two series machine1/exp_-jtheta3 ==
  dq_in : Inport
  Gain : Gain  Gain=2*Ts
  Gain1 : Gain
  MATLAB Function : MATLAB Function  TreatAsAtomicUnit=on
  y : Outport  PortDimensions=2
  wires:
  dq_in/1 -> MATLAB Function/1(u_dq)
  [w_e] -> Gain1/1
  Gain/1 -> MATLAB Function/2(theta)
  MATLAB Function/1(y) -> y/1
  Gain1/1 -> Gain/1

== system BIM_3phaseModel_MidInject_DPNV/Parallel DPNV/Current regulators for two series machine1/exp_-jtheta4 ==
  dq_in : Inport
  Gain : Gain  Gain=-Ts
  Gain1 : Gain  Gain=-1
  MATLAB Function : MATLAB Function  TreatAsAtomicUnit=on
  y : Outport  PortDimensions=2
  wires:
  dq_in/1 -> MATLAB Function/1(u_dq)
  [w_e] -> Gain1/1
  MATLAB Function/1(y) -> y/1
  Gain1/1 -> Gain/1
  Gain/1 -> MATLAB Function/2(theta)

== system BIM_3phaseModel_MidInject_DPNV/Parallel DPNV/Current regulators for two series machine1/exp_-jtheta5 ==
  dq_in : Inport
  Gain : Gain  Gain=2*Ts
  Gain1 : Gain  Gain=-1
  MATLAB Function : MATLAB Function  TreatAsAtomicUnit=on
  y : Outport  PortDimensions=2
  wires:
  dq_in/1 -> MATLAB Function/1(u_dq)
  [w_e] -> Gain1/1
  MATLAB Function/1(y) -> y/1
  Gain1/1 -> Gain/1
  Gain/1 -> MATLAB Function/2(theta)

== system BIM_3phaseModel_MidInject_DPNV/Parallel DPNV/Velocity Regulator/Scope4 ==
  1 : Inport
  2 : Inport  Port=2
  " 1 " : DataTypeConversion
  " 2 " : DataTypeConversion
  " InputMux " : Mux  Inputs=2
  " S-Function " : S-Function  FunctionName=plecs  SFunctionDeploymentMode=off  EnableBusSupport=off
  wires:
  " InputMux "/1 -> " S-Function "/1
  1/1 -> " 1 "/1
  " 1 "/1 -> " InputMux "/1
  2/1 -> " 2 "/1
  " 2 "/1 -> " InputMux "/2

== system BIM_3phaseModel_MidInject_DPNV/Parallel DPNV/Velocity Regulator/velocity regulator ==
  Err_v : Inport
  Delay1 : Delay  DelayLength=1  SampleTime=T
  Gain : Gain  Gain=Ctr_v_Ki*1
  Gain1 : Gain  Gain=Ctr_v_Kp*1
  Gain2 : Gain  Gain=Ts
  Scope1 : Subsystem  LoadFcn=plecs('sl', 300);  InitFcn=plecs('sl', 314);  StartFcn=plecs('sl', 308);  StopFcn=plecs('sl', 309);  mask{Settings=<binary blob, 232 chars, not shown>}
      mask init:
      | plecs('sl', 315);
      settings: CopyFcn=plecs('sl', 303);  DeleteFcn=plecs('sl', 305);  UndoDeleteFcn=plecs('sl', 306);  PreSaveFcn=plecs('sl', 311);  NameChangeFcn=plecs('sl', 310);  DestroyFcn=plecs('sl', 307);  OpenFcn=plecs('sl', 302);  ErrorFcn=plerrorfcn
      mask Display: plot([0.1 0.9 0.9 0.1 0.1], [0.9 0.9 0.5 0.5 0.9])
  Sum : Sum  Inputs=++|
  Sum4 : Sum  Inputs=|++
  Te* : Outport
  wires:
  Err_v/1 -> Scope1/1(1), Gain1/1, Gain/1
  Gain1/1 -> Sum/1
  Sum/1 -> Scope1/2(2), Te*/1
  Gain2/1 -> Sum4/1
  Gain/1 -> Gain2/1
  Sum4/1 -> Delay1/1, Sum/2
  Delay1/1 -> Sum4/2

== system BIM_3phaseModel_MidInject_DPNV/Parallel DPNV/XY Plot1/ InputMux  ==
  In1 : Inport
  In2 : Inport  Port=2
  Convert1 : DataTypeConversion
  Convert2 : DataTypeConversion
  Mux : Mux  Inputs=2
  Out : Outport
  wires:
  Convert2/1 -> Mux/2
  In2/1 -> Convert2/1
  Convert1/1 -> Mux/1
  In1/1 -> Convert1/1
  Mux/1 -> Out/1

== system BIM_3phaseModel_MidInject_DPNV/Mid Injection/Current regulators for two series machine1/Scope/ InputMux  ==
  In1 : Inport
  Convert1 : DataTypeConversion
  Mux : Mux  Inputs=1
  Out : Outport
  wires:
  Convert1/1 -> Mux/1
  In1/1 -> Convert1/1
  Mux/1 -> Out/1

== system BIM_3phaseModel_MidInject_DPNV/Mid Injection/Current regulators for two series machine1/Scope1/ InputMux  ==
  In1 : Inport
  Convert1 : DataTypeConversion
  Mux : Mux  Inputs=1
  Out : Outport
  wires:
  Convert1/1 -> Mux/1
  In1/1 -> Convert1/1
  Mux/1 -> Out/1

== system BIM_3phaseModel_MidInject_DPNV/Mid Injection/Current regulators for two series machine1/Scope2/ InputMux  ==
  In1 : Inport
  Convert1 : DataTypeConversion
  Mux : Mux  Inputs=1
  Out : Outport
  wires:
  Convert1/1 -> Mux/1
  In1/1 -> Convert1/1
  Mux/1 -> Out/1

== system BIM_3phaseModel_MidInject_DPNV/Mid Injection/Current regulators for two series machine1/Scope3/ InputMux  ==
  In1 : Inport
  Convert1 : DataTypeConversion
  Mux : Mux  Inputs=1
  Out : Outport
  wires:
  Convert1/1 -> Mux/1
  In1/1 -> Convert1/1
  Mux/1 -> Out/1

== system BIM_3phaseModel_MidInject_DPNV/Mid Injection/Current regulators for two series machine1/Scope5/ InputMux  ==
  In1 : Inport
  Convert1 : DataTypeConversion
  Mux : Mux  Inputs=1
  Out : Outport
  wires:
  Convert1/1 -> Mux/1
  In1/1 -> Convert1/1
  Mux/1 -> Out/1

== system BIM_3phaseModel_MidInject_DPNV/Mid Injection/Current regulators for two series machine1/Scope6/ InputMux  ==
  In1 : Inport
  Convert1 : DataTypeConversion
  Mux : Mux  Inputs=1
  Out : Outport
  wires:
  Convert1/1 -> Mux/1
  In1/1 -> Convert1/1
  Mux/1 -> Out/1

== system BIM_3phaseModel_MidInject_DPNV/Mid Injection/Current regulators for two series machine1/Scope7/ InputMux  ==
  In1 : Inport
  Convert1 : DataTypeConversion
  Mux : Mux  Inputs=1
  Out : Outport
  wires:
  Convert1/1 -> Mux/1
  In1/1 -> Convert1/1
  Mux/1 -> Out/1

== system BIM_3phaseModel_MidInject_DPNV/Mid Injection/Current regulators for two series machine1/XY Plot/ InputMux  ==
  In1 : Inport
  In2 : Inport  Port=2
  Convert1 : DataTypeConversion
  Convert2 : DataTypeConversion
  Mux : Mux  Inputs=2
  Out : Outport
  wires:
  Convert2/1 -> Mux/2
  In2/1 -> Convert2/1
  Convert1/1 -> Mux/1
  In1/1 -> Convert1/1
  Mux/1 -> Out/1

== system BIM_3phaseModel_MidInject_DPNV/Mid Injection/Current regulators for two series machine1/XY Plot1/ InputMux  ==
  In1 : Inport
  In2 : Inport  Port=2
  Convert1 : DataTypeConversion
  Convert2 : DataTypeConversion
  Mux : Mux  Inputs=2
  Out : Outport
  wires:
  Convert2/1 -> Mux/2
  In2/1 -> Convert2/1
  Convert1/1 -> Mux/1
  In1/1 -> Convert1/1
  Mux/1 -> Out/1

== system BIM_3phaseModel_MidInject_DPNV/Mid Injection/Velocity Regulator/velocity regulator/Scope1 ==
  1 : Inport
  2 : Inport  Port=2
  " 1 " : DataTypeConversion
  " 2 " : DataTypeConversion
  " InputMux " : Mux  Inputs=2
  " S-Function " : S-Function  FunctionName=plecs  SFunctionDeploymentMode=off  EnableBusSupport=off
  wires:
  " InputMux "/1 -> " S-Function "/1
  1/1 -> " 1 "/1
  " 1 "/1 -> " InputMux "/1
  2/1 -> " 2 "/1
  " 2 "/1 -> " InputMux "/2

== system BIM_3phaseModel_MidInject_DPNV/Parallel DPNV/Current regulators for two series machine1/Scope/ InputMux  ==
  In1 : Inport
  Convert1 : DataTypeConversion
  Mux : Mux  Inputs=1
  Out : Outport
  wires:
  Convert1/1 -> Mux/1
  In1/1 -> Convert1/1
  Mux/1 -> Out/1

== system BIM_3phaseModel_MidInject_DPNV/Parallel DPNV/Current regulators for two series machine1/Scope1/ InputMux  ==
  In1 : Inport
  Convert1 : DataTypeConversion
  Mux : Mux  Inputs=1
  Out : Outport
  wires:
  Convert1/1 -> Mux/1
  In1/1 -> Convert1/1
  Mux/1 -> Out/1

== system BIM_3phaseModel_MidInject_DPNV/Parallel DPNV/Current regulators for two series machine1/Scope2/ InputMux  ==
  In1 : Inport
  Convert1 : DataTypeConversion
  Mux : Mux  Inputs=1
  Out : Outport
  wires:
  Convert1/1 -> Mux/1
  In1/1 -> Convert1/1
  Mux/1 -> Out/1

== system BIM_3phaseModel_MidInject_DPNV/Parallel DPNV/Current regulators for two series machine1/Scope3/ InputMux  ==
  In1 : Inport
  Convert1 : DataTypeConversion
  Mux : Mux  Inputs=1
  Out : Outport
  wires:
  Convert1/1 -> Mux/1
  In1/1 -> Convert1/1
  Mux/1 -> Out/1

== system BIM_3phaseModel_MidInject_DPNV/Parallel DPNV/Current regulators for two series machine1/Scope5/ InputMux  ==
  In1 : Inport
  Convert1 : DataTypeConversion
  Mux : Mux  Inputs=1
  Out : Outport
  wires:
  Convert1/1 -> Mux/1
  In1/1 -> Convert1/1
  Mux/1 -> Out/1

== system BIM_3phaseModel_MidInject_DPNV/Parallel DPNV/Current regulators for two series machine1/Scope6/ InputMux  ==
  In1 : Inport
  Convert1 : DataTypeConversion
  Mux : Mux  Inputs=1
  Out : Outport
  wires:
  Convert1/1 -> Mux/1
  In1/1 -> Convert1/1
  Mux/1 -> Out/1

== system BIM_3phaseModel_MidInject_DPNV/Parallel DPNV/Current regulators for two series machine1/Scope7/ InputMux  ==
  In1 : Inport
  Convert1 : DataTypeConversion
  Mux : Mux  Inputs=1
  Out : Outport
  wires:
  Convert1/1 -> Mux/1
  In1/1 -> Convert1/1
  Mux/1 -> Out/1

== system BIM_3phaseModel_MidInject_DPNV/Parallel DPNV/Current regulators for two series machine1/XY Plot/ InputMux  ==
  In1 : Inport
  In2 : Inport  Port=2
  Convert1 : DataTypeConversion
  Convert2 : DataTypeConversion
  Mux : Mux  Inputs=2
  Out : Outport
  wires:
  Convert2/1 -> Mux/2
  In2/1 -> Convert2/1
  Convert1/1 -> Mux/1
  In1/1 -> Convert1/1
  Mux/1 -> Out/1

== system BIM_3phaseModel_MidInject_DPNV/Parallel DPNV/Current regulators for two series machine1/XY Plot1/ InputMux  ==
  In1 : Inport
  In2 : Inport  Port=2
  Convert1 : DataTypeConversion
  Convert2 : DataTypeConversion
  Mux : Mux  Inputs=2
  Out : Outport
  wires:
  Convert2/1 -> Mux/2
  In2/1 -> Convert2/1
  Convert1/1 -> Mux/1
  In1/1 -> Convert1/1
  Mux/1 -> Out/1

== system BIM_3phaseModel_MidInject_DPNV/Parallel DPNV/Velocity Regulator/velocity regulator/Scope1 ==
  1 : Inport
  2 : Inport  Port=2
  " 1 " : DataTypeConversion
  " 2 " : DataTypeConversion
  " InputMux " : Mux  Inputs=2
  " S-Function " : S-Function  FunctionName=plecs  SFunctionDeploymentMode=off  EnableBusSupport=off
  wires:
  " InputMux "/1 -> " S-Function "/1
  1/1 -> " 1 "/1
  " 1 "/1 -> " InputMux "/1
  2/1 -> " 2 "/1
  " 2 "/1 -> " InputMux "/2

== matlab function BIM_3phaseModel_MidInject_DPNV/Mid Injection/Current regulators for two series machine1/exp_-jtheta2/MATLAB Function ==
  data: u_dq input; y output; theta input
function y = exp_jtheta(u_dq, theta)
u_d = u_dq(1);
u_q = u_dq(2);
y_d = cos(theta)*u_d - sin(theta)*u_q;
y_q = sin(theta)*u_d + cos(theta)*u_q;
y = [y_d y_q];
% y(1) = y_d;
% y(2) = y_q;

== matlab function BIM_3phaseModel_MidInject_DPNV/Mid Injection/Current regulators for two series machine1/exp_-jtheta3/MATLAB Function ==
  data: u_dq input; y output; theta input
function y = exp_jtheta(u_dq, theta)
u_d = u_dq(1);
u_q = u_dq(2);
y_d = cos(theta)*u_d - sin(theta)*u_q;
y_q = sin(theta)*u_d + cos(theta)*u_q;
y = [y_d y_q];

== matlab function BIM_3phaseModel_MidInject_DPNV/Parallel DPNV/Current regulators for two series machine1/exp_-jtheta2/MATLAB Function ==
  data: u_dq input; y output; theta input
function y = exp_jtheta(u_dq, theta)
u_d = u_dq(1);
u_q = u_dq(2);
y_d = cos(theta)*u_d - sin(theta)*u_q;
y_q = sin(theta)*u_d + cos(theta)*u_q;
y = [y_d y_q];
% y(1) = y_d;
% y(2) = y_q;

== matlab function BIM_3phaseModel_MidInject_DPNV/Parallel DPNV/Current regulators for two series machine1/exp_-jtheta3/MATLAB Function ==
  data: u_dq input; y output; theta input
function y = exp_jtheta(u_dq, theta)
u_d = u_dq(1);
u_q = u_dq(2);
y_d = cos(theta)*u_d - sin(theta)*u_q;
y_q = sin(theta)*u_d + cos(theta)*u_q;
y = [y_d y_q];

== matlab function BIM_3phaseModel_MidInject_DPNV/Parallel DPNV/Current regulators for two series machine1/exp_-jtheta4/MATLAB Function ==
  data: u_dq input; y output; theta input
function y = exp_jtheta(u_dq, theta)
u_d = u_dq(1);
u_q = u_dq(2);
y_d = cos(theta)*u_d - sin(theta)*u_q;
y_q = sin(theta)*u_d + cos(theta)*u_q;
y = [y_d y_q];

== matlab function BIM_3phaseModel_MidInject_DPNV/Parallel DPNV/Current regulators for two series machine1/exp_-jtheta5/MATLAB Function ==
  data: u_dq input; y output size=[1 2]; theta input
function y = exp_jtheta(u_dq, theta)
u_d = u_dq(1);
u_q = u_dq(2);
y_d = cos(theta)*u_d - sin(theta)*u_q;
y_q = sin(theta)*u_d + cos(theta)*u_q;
y = [y_d y_q];

== matlab function BIM_3phaseModel_MidInject_DPNV/Mid Injection/Current regulators for two series machine1/exp_-jtheta4/MATLAB Function ==
  data: u_dq input; y output; theta input
function y = exp_jtheta(u_dq, theta)
u_d = u_dq(1);
u_q = u_dq(2);
y_d = cos(theta)*u_d - sin(theta)*u_q;
y_q = sin(theta)*u_d + cos(theta)*u_q;
y = [y_d y_q];

== matlab function BIM_3phaseModel_MidInject_DPNV/Mid Injection/Current regulators for two series machine1/exp_-jtheta5/MATLAB Function ==
  data: u_dq input; y output size=[1 2]; theta input
function y = exp_jtheta(u_dq, theta)
u_d = u_dq(1);
u_q = u_dq(2);
y_d = cos(theta)*u_d - sin(theta)*u_q;
y_q = sin(theta)*u_d + cos(theta)*u_q;
y = [y_d y_q];

== matlab function BIM_3phaseModel_MidInject_DPNV/Parallel DPNV/UFO2/Reference Calculation ==
  data: Te_star input; lam_dr_er_star input; i_qs_er_star output; w_sl_star output; L_m input; tau_r input
function [i_qs_er_star, w_sl_star]  = SlipCalc(Te_star, lam_dr_er_star, L_m, tau_r)

if lam_dr_er_star == 0
    i_qs_er_star = 0;
    w_sl_star = 0;
else 
    i_qs_er_star = Te_star/lam_dr_er_star;
    w_sl_star = L_m*i_qs_er_star/(tau_r*lam_dr_er_star);
end

== matlab function BIM_3phaseModel_MidInject_DPNV/Mid Injection/UFO2/Reference Calculation ==
  data: Te_star input; lam_dr_er_star input; i_qs_er_star output; w_sl_star output; L_m input; tau_r input
function [i_qs_er_star, w_sl_star]  = SlipCalc(Te_star, lam_dr_er_star, L_m, tau_r)

if lam_dr_er_star == 0
    i_qs_er_star = 0;
    w_sl_star = 0;
else 
    i_qs_er_star = Te_star/lam_dr_er_star;
    w_sl_star = L_m*i_qs_er_star/(tau_r*lam_dr_er_star);
end
